simulink model "quad_control"  (R2023b)
settings: Solver=ode3  StartTime=0.0  StopTime=100  FixedStep=0.01  RelTol=1e-3  EnableMultiTasking=on
values from neighbouring files (symbols this model uses):
  g = 9.8    [init2.m]
  m = 0.18    [init2.m]
undefined symbols (not defined in the file or in its folder): attitude_control, model, position_control, sliding_var
libraries: simulink x2
settings Model: Creator=smishra  LastModifiedBy=manah
settings SolverCC: AlgebraicLoopSolver=TrustRegion
settings DataIOCC: LimitDataPoints=on  SaveFormat=Array  ReturnWorkspaceOutputs=off  Refine=5
settings OptimizationCC: LifeSpan=inf
settings DebuggingCC: UnconnectedInputMsg=warning  UnconnectedOutputMsg=warning  UnconnectedLineMsg=warning  SFUnexpectedBacktrackingDiag=warning  SFNoUnconditionalDefaultTransitionDiag=warning  SFExecutionAtInitializationDiag=none  ArithmeticOperatorsInVariantConditions=warning
settings HardwareCC: ProdBitPerPointer=32  ProdBitPerSizeT=32  ProdBitPerPtrDiffT=32  ProdLargestAtomicFloat=None  ProdIntDivRoundTo=Undefined  ProdEndianess=Unspecified  ProdWordSize=32  ProdHWDeviceType=32-bit Generic
settings ModelReferenceCC: PropagateSignalLabelsOutOfModel=off
settings SFSimCC: SimUseLocalCustomCode=off  CustomCodeUndefinedFunction=UseInterfaceOnly
settings RTWCC: RTWUseLocalCustomCode=off
settings CodeAppCC: StateflowObjectComments=on
settings GRTTargetCC: TargetLangStandard=C89/C90 (ANSI)
settings ConfigComp: CovMetricSettings=dw  CovSaveCumulativeToWorkspaceVar=on  CovSaveSingleToWorkspaceVar=on  CovExternalEMLEnable=off

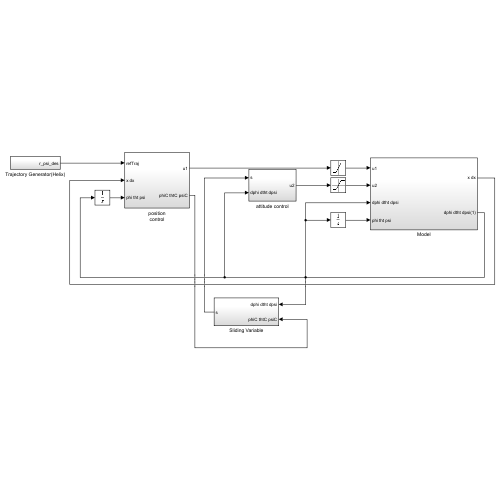
[thumbnail: Simulink's stored preview of the top-level diagram]
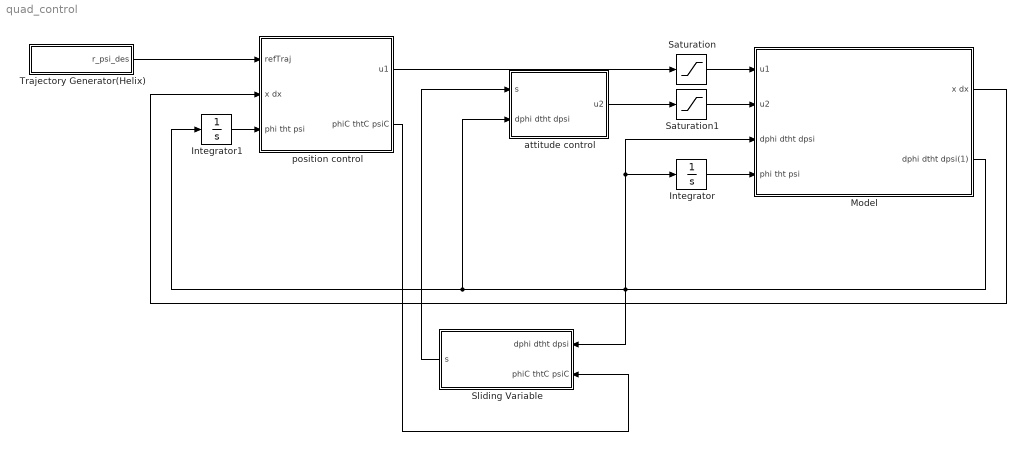
== system quad_control ==
  Integrator : Integrator
  Integrator1 : Integrator
  Model : Subsystem
  Saturation : Saturate  UpperLimit=2*m*g  LowerLimit=0
  Saturation1 : Saturate  UpperLimit=0.2  LowerLimit=-0.2
  Sliding Variable : Subsystem
  Trajectory Generator(Helix) : Subsystem
  attitude control : Subsystem
  position control : Subsystem
  wires:
  Trajectory Generator(Helix)/1(r_psi_des) -> position control/1(refTraj)
  Model/2(dphi dtht dpsi(1)) -> Integrator1/1, attitude control/2(dphi dtht dpsi), Sliding Variable/1(dphi dtht dpsi), Model/3(dphi dtht dpsi), Integrator/1
  Integrator/1 -> Model/4(phi tht psi)
  Integrator1/1 -> position control/3(phi tht psi)
  Model/1(x dx) -> position control/2(x dx)
  Sliding Variable/1(s) -> attitude control/1(s)
  position control/2(phiC thtC psiC) -> Sliding Variable/2(phiC thtC psiC)
  Saturation/1 -> Model/1(u1)
  position control/1(u1) -> Saturation/1
  attitude control/1(u2) -> Saturation1/1
  Saturation1/1 -> Model/2(u2)

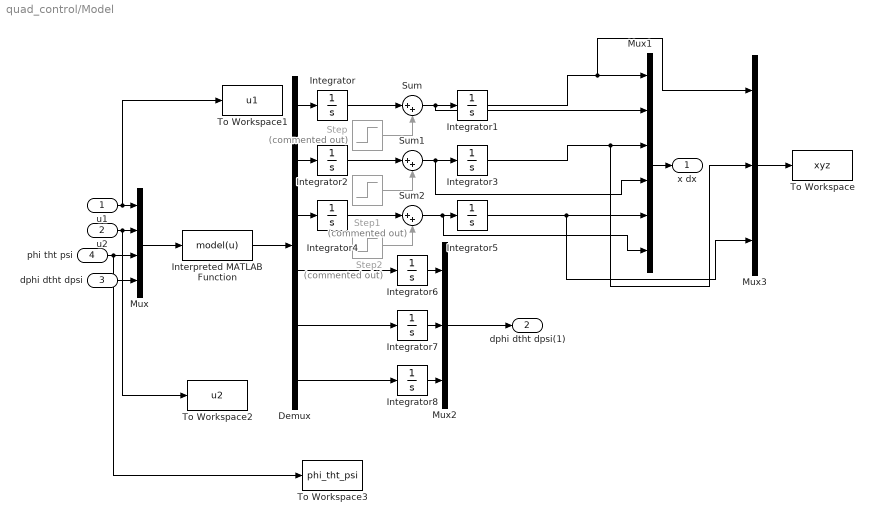
== system quad_control/Model ==
  u1 : Inport
  u2 : Inport  Port=2
  dphi dtht dpsi : Inport  Port=3
  phi tht psi : Inport  Port=4
  Demux : Demux  Outputs=6
  Integrator{,1..2,4,6..8} (7 alike) : Integrator
  Integrator3 : Integrator  InitialCondition=8
  Integrator5 : Integrator  InitialCondition=-8
  Interpreted MATLAB Function : MATLABFcn  MATLABFcn=model(u)  OutputDimensions=6
  Mux : Mux
  Mux1 : Mux  Inputs=6
  Mux2 : Mux  Inputs=3
  Mux3 : Mux  Inputs=3
  Step : Step  Commented=on  Time=25  After=5  SampleTime=0
  Step1 : Step  Commented=on  Time=25  After=5  SampleTime=0
  Step2 : Step  Commented=on  Time=25  After=5  SampleTime=0
  Sum : Sum  Inputs=|++
  Sum1 : Sum  Inputs=|++
  Sum2 : Sum  Inputs=|++
  To Workspace : ToWorkspace  VariableName=xyz  SampleTime=-1
  To Workspace1 : ToWorkspace  VariableName=u1  SampleTime=-1
  To Workspace2 : ToWorkspace  VariableName=u2  SampleTime=-1
  To Workspace3 : ToWorkspace  VariableName=phi_tht_psi  SampleTime=-1
  x dx : Outport
  dphi dtht dpsi(1) : Outport  Port=2
  wires:
  Integrator5/1 -> Mux3/3, Mux1/5
  Mux2/1 -> dphi dtht dpsi(1)/1
  Mux1/1 -> x dx/1
  Mux/1 -> Interpreted MATLAB Function/1
  Integrator3/1 -> Mux3/2, Mux1/3
  Demux/3 -> Integrator4/1
  Demux/1 -> Integrator/1
  Integrator1/1 -> Mux3/1, Mux1/1
  Integrator7/1 -> Mux2/2
  Interpreted MATLAB Function/1 -> Demux/1
  Integrator8/1 -> Mux2/3
  Demux/2 -> Integrator2/1
  Integrator6/1 -> Mux2/1
  phi tht psi/1 -> Mux/3, To Workspace3/1
  Mux3/1 -> To Workspace/1
  u1/1 -> To Workspace1/1, Mux/1
  u2/1 -> To Workspace2/1, Mux/2
  dphi dtht dpsi/1 -> Mux/4
  Demux/4 -> Integrator6/1
  Demux/5 -> Integrator7/1
  Demux/6 -> Integrator8/1
  Integrator/1 -> Sum/1
  Sum/1 -> Mux1/2, Integrator1/1
  Integrator2/1 -> Sum1/1
  Sum1/1 -> Mux1/4, Integrator3/1
  Integrator4/1 -> Sum2/1
  Sum2/1 -> Mux1/6, Integrator5/1
  Step/1 -> Sum/2
  Step1/1 -> Sum1/2
  Step2/1 -> Sum2/2

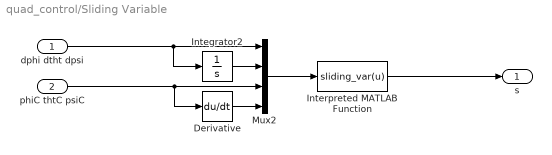
== system quad_control/Sliding Variable ==
  dphi dtht dpsi : Inport
  phiC thtC psiC : Inport  Port=2
  Derivative : Derivative
  Integrator2 : Integrator
  Interpreted MATLAB Function : MATLABFcn  MATLABFcn=sliding_var(u)  OutputDimensions=3
  Mux2 : Mux
  s : Outport
  wires:
  Integrator2/1 -> Mux2/2
  Mux2/1 -> Interpreted MATLAB Function/1
  dphi dtht dpsi/1 -> Integrator2/1, Mux2/1
  Interpreted MATLAB Function/1 -> s/1
  phiC thtC psiC/1 -> Derivative/1, Mux2/3
  Derivative/1 -> Mux2/4

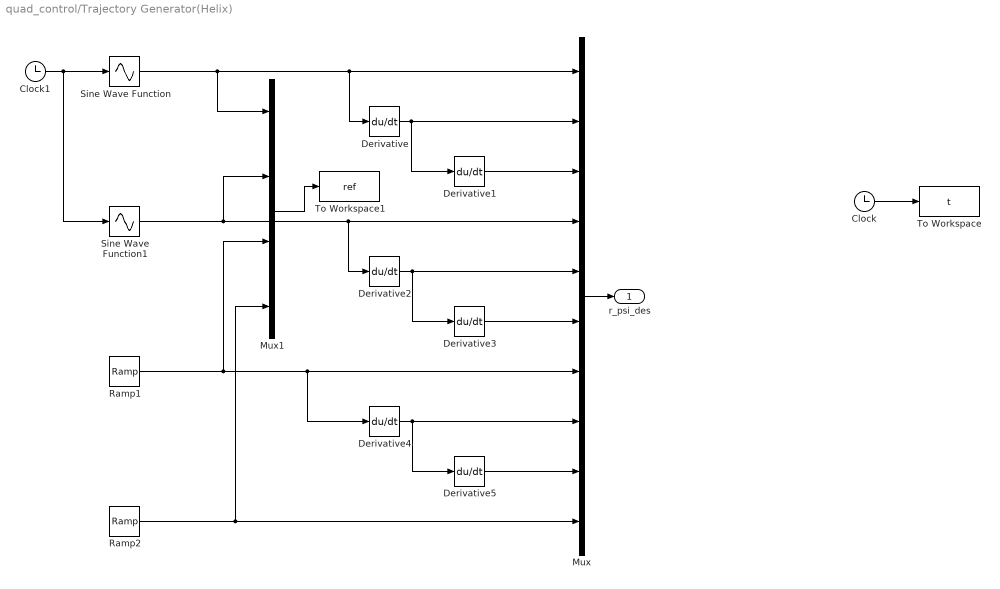
== system quad_control/Trajectory Generator(Helix) ==
  Clock : Clock
  Clock1 : Clock
  Derivative{,1..5} (6 alike) : Derivative
  Mux : Mux  Inputs=10
  Mux1 : Mux
  Ramp1 : simulink/Sources/Ramp  slope=0.2  start=0  InitialOutput=-8
  Ramp2 : simulink/Sources/Ramp  slope=0  start=0  InitialOutput=0
  Sine Wave Function : Sin  TimeSource=Use external signal  Amplitude=8  Frequency=0.1  SampleTime=0
  Sine Wave Function1 : Sin  TimeSource=Use external signal  Amplitude=8  Frequency=0.1  Phase=pi/2  SampleTime=0
  To Workspace : ToWorkspace  VariableName=t  SampleTime=-1
  To Workspace1 : ToWorkspace  VariableName=ref  SampleTime=-1
  r_psi_des : Outport
  wires:
  Derivative2/1 -> Mux/5, Derivative3/1
  Derivative4/1 -> Mux/8, Derivative5/1
  Derivative/1 -> Mux/2, Derivative1/1
  Derivative1/1 -> Mux/3
  Derivative3/1 -> Mux/6
  Derivative5/1 -> Mux/9
  Sine Wave Function/1 -> Mux1/1, Mux/1, Derivative/1
  Ramp2/1 -> Mux1/4, Mux/10
  Mux/1 -> r_psi_des/1
  Clock/1 -> To Workspace/1
  Clock1/1 -> Sine Wave Function1/1, Sine Wave Function/1
  Ramp1/1 -> Mux1/3, Derivative4/1, Mux/7
  Mux1/1 -> To Workspace1/1
  Sine Wave Function1/1 -> Mux1/2, Derivative2/1, Mux/4

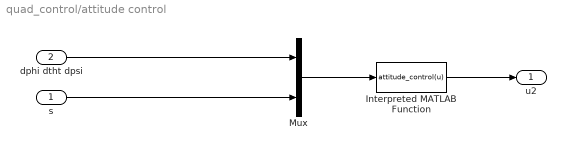
== system quad_control/attitude control ==
  s : Inport
  dphi dtht dpsi : Inport  Port=2
  Interpreted MATLAB Function : MATLABFcn  MATLABFcn=attitude_control(u)  OutputDimensions=3
  Mux : Mux  Inputs=2
  u2 : Outport
  wires:
  Mux/1 -> Interpreted MATLAB Function/1
  Interpreted MATLAB Function/1 -> u2/1
  dphi dtht dpsi/1 -> Mux/1
  s/1 -> Mux/2

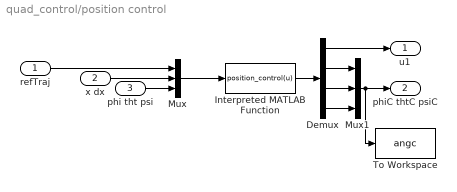
== system quad_control/position control ==
  refTraj : Inport
  x dx : Inport  Port=2
  phi tht psi : Inport  Port=3
  Demux : Demux
  Interpreted MATLAB Function : MATLABFcn  MATLABFcn=position_control(u)  OutputDimensions=4
  Mux : Mux  Inputs=3
  Mux1 : Mux  Inputs=3
  To Workspace : ToWorkspace  VariableName=angc  SampleTime=-1
  u1 : Outport
  phiC thtC psiC : Outport  Port=2
  wires:
  Mux/1 -> Interpreted MATLAB Function/1
  refTraj/1 -> Mux/1
  x dx/1 -> Mux/2
  phi tht psi/1 -> Mux/3
  Interpreted MATLAB Function/1 -> Demux/1
  Demux/1 -> u1/1
  Demux/2 -> Mux1/1
  Demux/3 -> Mux1/2
  Demux/4 -> Mux1/3
  Mux1/1 -> To Workspace/1, phiC thtC psiC/1
